simulink model "tflight"  (R2021a)
settings: Solver=VariableStepAuto  StartTime=0.0  StopTime=300  RelTol=1e-3
settings Model: EnablePacing=on  PacingRate=3  Creator=kasra  LastModifiedBy=kasra
settings SolverCC: AlgebraicLoopSolver=TrustRegion
settings DebuggingCC: SFMachineParentedDataDiag=warning

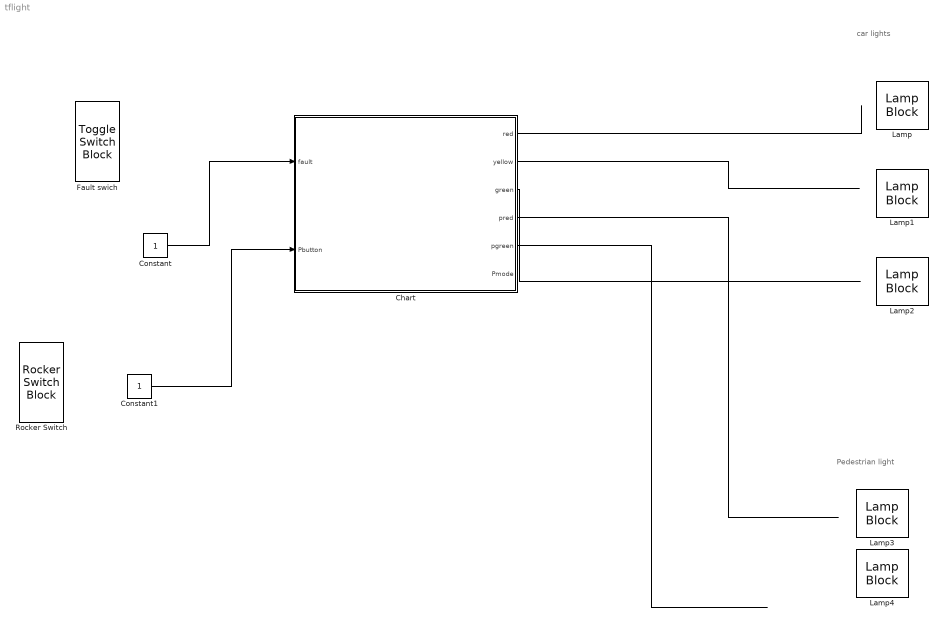
== system tflight ==
  note: Pedestrian light
  note: car lights
  Chart : Stateflow chart  TreatAsAtomicUnit=on
  Constant : Constant
  Constant1 : Constant
  Fault swich : ToggleSwitchBlock  Description=Fault switch
      settings: Values={{'Off', 'On'}, [0 1]}
  Lamp{,1..4} (5 alike) : LampBlock
  Rocker Switch : RockerSwitchBlock
      settings: Values={{'Off', 'On'}, [0 1]}
  wires:
  Chart/2(yellow) -> ?
  Chart/3(green) -> ?
  Constant/1 -> Chart/1(fault)
  Chart/1(red) -> ?
  Chart/4(pred) -> ?
  Chart/5(pgreen) -> ?
  Constant1/1 -> Chart/2(Pbutton)

== stateflow chart tflight/Chart ==
  state Norm
    state Pstop
      entry:
      red = 0;
      yellow = 1;
      green= 0;
    state Go
      entry:
      red = 0;
      yellow = 0;
      green= 1;
    state Stop
      entry:
      red = 1;
      yellow = 0;
      green= 0;
    state Initial_state
      entry:
      red = 0;
      yellow = 0;
      green= 0;
      Pmode = 0;
      pred = 1;
      pgreen = 0
    state Pmode2
      entry :
      Pmode = 1;
      pred = 1;
      pgreen = 0;
    state pStop
      entry :
      pred = 1;
      pgreen = 0;
      Pmode = 0;
    state pGo
      entry:
      pred = 0;
      pgreen = 1;
      green = 0;
      yellow = 0;
      red = 1;
    (default) -> Initial_state
    Initial_state -> Norm.Stop [order 1] : after(1,sec)
    (junction 163) -> Norm.Stop [order 2] : [Pmode == 0]
    (junction 138) -> Go [order 1] : after(10,sec)
    (junction 164) -> Pstop : [Pmode == 0]
    Pstop -> (junction 163) : after(2,sec)
    (junction 163) -> (junction 160) [order 1] : {Pbutton == 1}
    Go -> (junction 164) : after(30,sec)
    Initial_state -> Pmode2 [order 2] : [Pbutton == 1]
    Norm.Stop -> (junction 138) : [Pmode ==0]
    pStop -> Go : after(2,sec)
    (junction 138) -> (junction 160) [order 2] : {Pbutton == 1}
    (junction 160) -> Pmode2 : [Pbutton ==1]
    pGo -> pStop : after(10,sec)
    Pmode2 -> pGo : after(10,sec)
  state Decidestate
  state faultstate
    state Stop
      entry:
      red = 0;
      yellow = 0;
      green= 0;
      pred = 0;
    state F2
      entry:
      yellow= 1
    (default) -> faultstate.Stop
    F2 -> faultstate.Stop : after(1,sec)
    faultstate.Stop -> F2 : after(1,sec)
  Decidestate -> (junction 113) [order 1] : [fault == 0]
  (junction 113) -> Norm
  (default) -> Decidestate
  Decidestate -> faultstate [order 2] : [fault == 1]
  faultstate -> Norm : [fault == 0]
  Norm -> faultstate : [fault == 1]
  data: red output; yellow output; green output; fault input; pred output; pgreen output; Pbutton input; Pmode output double =0
